simulink model "VectorControl002"  (R2018a)
settings: Solver=ode15s  StartTime=0  StopTime=1  FixedStep=0.001  MaxStep=1e-4  RelTol=1e-6  AbsTol=1e-6  EnableMultiTasking=on
PreLoadFcn:
  | Param000
StopFcn:
  | % TNAnalyzexxxPlot
values from neighbouring files (symbols this model uses):
  DCVoltage = 100    [Param000.m]    (also in StartSim.m; StartSim_NoNoise.m)
  MotInertia = 10*rand()*1e-3    [Param000.m]    (also in StartSim.m = 0.1*rand()*1e-3; StartSim_NoNoise.m = 0.1*rand()*1e-3)
  MotPhaseL = 0.01 + 100 * rand()    [Param000.m]    (also in StartSim.m = (0.001 + 10 * rand())*1e-3; StartSim_NoNoise.m = (0.001 + 10 * rand())*1e-3)
  MotPhaseR = 0.01 + 100 * rand()    [Param000.m]    (also in StartSim.m = 0.001 + 10 * rand(); StartSim_NoNoise.m = 0.001 + 10 * rand())
  MotPole = 20    [Param000.m]    (also in StartSim.m = 1; StartSim_NoNoise.m = 1)
  MotVisco = rand()*1e-6    [Param000.m]    (also in StartSim.m = 0.01*rand()*1e-6; StartSim_NoNoise.m = 0.01*rand()*1e-6)
  Ts = 1e-6    (= 1e-06)    [StartSim.m]    (also in StartSim_NoNoise.m)
undefined symbols (not defined in the file or in its folder): AmpCap, AmpCapR, MotLineR, PowerLineR
libraries: powerlib x43, simulink x2, powerlib_meascontrol x2, pePwmGeneratorTwoLevel x1
Description:
  | This example illustrates use of the BLDC in a closed-loop
  | speed and voltage control on a 1 kW, 3000 rpm industrial motor
  | 
  | 
  | Copyright 2008-2017 The MathWorks, Inc.
settings Model: ExtModeAutoUpdateStatusClock=off  Creator=MathWorks  LastModifiedBy=1468993
settings SolverCC: AutoScaleAbsTol=off  MaxConsecutiveZCs=10000  ZeroCrossAlgorithm=Adaptive  DecoupledContinuousIntegration=on
settings DataIOCC: Decimation=100  SaveFormat=Array  ReturnWorkspaceOutputs=on  SignalLoggingName=sigsOut
settings OptimizationCC: DefaultParameterBehavior=Inlined  UseDivisionForNetSlopeComputation=on  UseFloatMulNetSlope=on  InlineInvariantSignals=on  PassReuseOutputArgsAs=Individual arguments  ExpressionDepthLimit=2147483647  ZeroExternalMemoryAtStartup=off  ZeroInternalMemoryAtStartup=off  NoFixptDivByZeroProtection=on  EfficientFloat2IntCast=on  LifeSpan=1  OptimizeDataStoreBuffers=off  BusAssignmentInplaceUpdate=off  OptimizationLevel=level0
settings DebuggingCC: AlgebraicLoopMsg=none  UnderspecifiedInitializationDetection=Classic  MergeDetectMultiDrivingBlocksExec=none  SignalResolutionControl=TryResolveAllWithWarning  MultiTaskDSMMsg=warning  MultiTaskCondExecSysMsg=none  ParameterTunabilityLossMsg=error  FcnCallInpInsideContextMsg=warning  StateNameClashWarn=warning  SFUnexpectedBacktrackingDiag=warning  SFNoUnconditionalDefaultTransitionDiag=warning  SFExecutionAtInitializationDiag=none
settings HardwareCC: ProdBitPerPointer=32  ProdBitPerSizeT=32  ProdBitPerPtrDiffT=32  ProdLargestAtomicInteger=Long  ProdWordSize=32  ProdLongLongMode=on  ProdHWDeviceType=ARM Compatible->ARM 10  TargetUnknown=on
settings ModelReferenceCC: PropagateSignalLabelsOutOfModel=off
settings SFSimCC: MATLABDynamicMemAlloc=off
settings RTWCC: SystemTargetFile=ert.tlc  TemplateMakefile=ert_default_tmf  GenerateReport=on  IncludeHyperlinkInReport=on  LaunchReport=on  GenerateTraceInfo=on  GenerateTraceReport=on  GenerateTraceReportSl=on  GenerateTraceReportSf=on  GenerateTraceReportEml=on  GenerateCodeMetricsReport=on
settings CodeAppCC: ForceParamTrailComments=on  IgnoreCustomStorageClasses=off  OperatorAnnotations=on  SimulinkDataObjDesc=on  SFDataObjDesc=on  CustomSymbolStrGlobalVar=rt$N$M  CustomSymbolStrType=$N$M  CustomSymbolStrFcn=$N$M$F  CustomSymbolStrMacro=$N$M  InsertBlockDesc=on
settings ERTTargetCC: GenerateSampleERTMain=on  IncludeMdlTerminateFcn=off  CombineSignalStateStructs=on  SupportComplex=off  SupportContinuousTime=on  SupportNonInlinedSFcns=on  InlinedParameterPlacement=NonHierarchical  ERTCustomFileTemplate=example_file_process.tlc  ERTFilePackagingFormat=CompactWithDataFile
settings ConfigComp: CovMetricSettings=dw  CovHtmlReporting=on  CovSaveCumulativeToWorkspaceVar=on  CovSaveSingleToWorkspaceVar=on  CovExternalEMLEnable=off  CovSFcnEnable=off
settings SimscapeCC: SimscapeNormalizeSystem=off

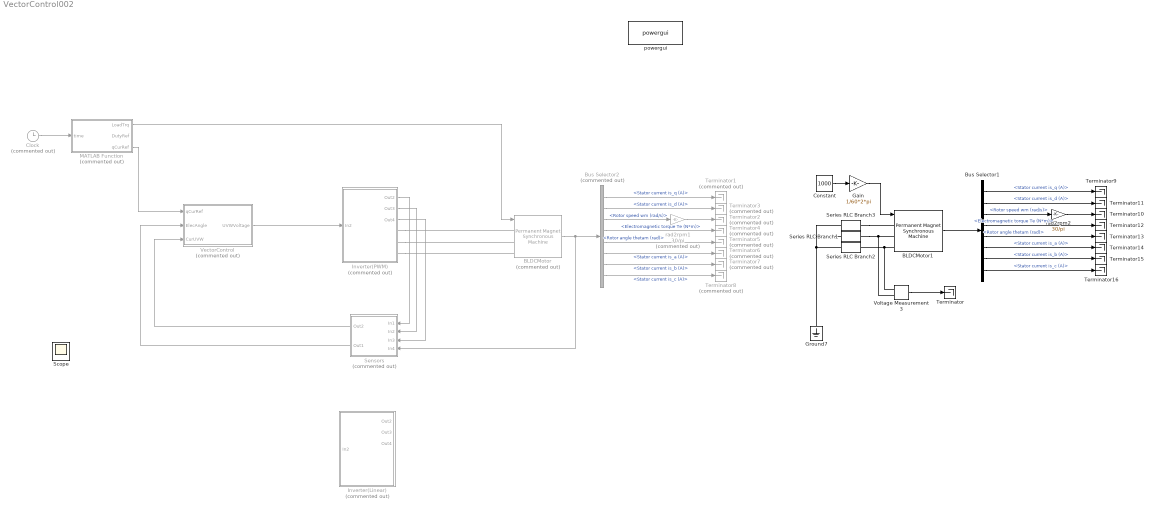
== system VectorControl002 ==
  BLDCMotor : powerlib/Machines/Permanent Magnet Synchronous Machine  Commented=on  NbPhases=3  FluxDistribution=Sinusoidal  RotorType=Round  MechanicalLoad=Torque Tm  PresetModel=No  ShowDetailedParameters=on  MeasurementBus=off  Resistance=MotPhaseR  Inductance=MotPhaseL  dqInductances=[8.5e-3, 8.5e-3]  La=MotPhaseL  MachineConstant=Voltage Constant (V_peak L-L / krpm)  Flux=0.01021  VoltageCst=MotVoltageConst  TorqueCst=0.30629  Flat=120  Mechanical=[MotInertia MotVisco MotPole 0]  PolePairs=20  InitialConditions=[0,0, 0,0]  InitialConditions5ph=[0 0 0 0 0 0]  TsPowergui=0  TsBlock=-1  RefAngle=90 degrees behind phase A axis (modified Park)
      settings: SourceProductName=Simscape Power Systems
  BLDCMotor1 : powerlib/Machines/Permanent Magnet Synchronous Machine  NbPhases=3  FluxDistribution=Sinusoidal  RotorType=Round  MechanicalLoad=Speed w  PresetModel=No  ShowDetailedParameters=on  MeasurementBus=off  Resistance=MotPhaseR  Inductance=MotPhaseL  dqInductances=[8.5e-3, 8.5e-3]  La=MotPhaseL  MachineConstant=Voltage Constant (V_peak L-L / krpm)  Flux=0.01021  VoltageCst=MotVoltageConst  TorqueCst=0.30629  Flat=120  Mechanical=[MotInertia MotVisco MotPole 0]  PolePairs=20  InitialConditions=[0,0, 0,0]  InitialConditions5ph=[0 0 0 0 0 0]  TsPowergui=0  TsBlock=-1  RefAngle=90 degrees behind phase A axis (modified Park)
      settings: SourceProductName=Simscape Power Systems
  Bus Selector1 : BusSelector  OutputSignals=Stator current is_q (A),Stator current is_d (A),Rotor speed wm (rad/s),Electromagnetic torque Te (N*m),Rotor angle thetam (rad),Stator current is_a (A),Stator current is_b (A),Stator current is_c (A)
  Bus Selector2 : BusSelector  Commented=on  OutputSignals=Stator current is_q (A),Stator current is_d (A),Rotor speed wm (rad/s),Electromagnetic torque Te (N*m),Rotor angle thetam (rad),Stator current is_a (A),Stator current is_b (A),Stator current is_c (A)
  Clock : Clock  Commented=on
  Constant : Constant  Value=1000
  Gain : Gain  Gain=1/60*2*pi
  Ground7 : powerlib/Elements/Ground  LConnTagsString=a
  Inverter(Linear) : Subsystem  Commented=on
  Inverter(PWM) : Subsystem  Commented=on
  MATLAB Function : MATLAB Function  Commented=on  TreatAsAtomicUnit=on
  Sensors : Subsystem  Commented=on
  Series RLC Branch1 : powerlib/Elements/Series RLC Branch  LConnTagsString=__new0  RConnTagsString=__new0  BranchType=R  Resistance=1e6  Inductance=1e-3  SetiL0=off  InitialCurrent=0  Capacitance=100e-6  Setx0=on  InitialVoltage=3.7*7*3  Measurements=None
  Series RLC Branch2 : powerlib/Elements/Series RLC Branch  LConnTagsString=__new0  RConnTagsString=__new0  BranchType=R  Resistance=1e6  Inductance=1e-3  SetiL0=off  InitialCurrent=0  Capacitance=100e-6  Setx0=on  InitialVoltage=3.7*7*3  Measurements=None
  Series RLC Branch3 : powerlib/Elements/Series RLC Branch  LConnTagsString=__new0  RConnTagsString=__new0  BranchType=R  Resistance=1e6  Inductance=1e-3  SetiL0=off  InitialCurrent=0  Capacitance=100e-6  Setx0=on  InitialVoltage=3.7*7*3  Measurements=None
  Terminator{,9..16} (9 alike) : Terminator
  Terminator{1..8} (8 alike) : Terminator  Commented=on
  VectorControl : Subsystem  Commented=on
  Voltage Measurement3 : powerlib/Measurements/Voltage Measurement  PhasorSimulation=off  OutputType=Complex  PSBequivalent=0
  powergui : powerlib/powergui  Priority=2  SimulationMode=Continuous  SampleTime=Ts  frequency=60  Iterations=50  frequencyindice=0  Pbase=100e6  ErrMax=1e-4  UnitsV=kV  UnitsW=MW  buscounter=0  FunctionMessages=off  echomessages=off  EnableUseOfTLC=off  CurrentSourceSwitches=off  DisableSnubberDevices=off  DisableRonSwitches=off  DisableVfSwitches=off  DisplayEquations=off  SolverType=Tustin/Backward Euler (TBE)  Interpol=off  ExternalGateDelay=off  methode=off  Ts=100  x0status=blocks  SPID=off  SwTol=0  HookPort=off  RestoreLinks=warning  ResistiveCurrentMeasurement=off  Frange=[0:2:500]  Ylog=off  Xlog=on  ShowGrid=off  save=off  variable=ZData  structure=0  ZoomFFT=on  StartTime=0.0  cycles=1  DisplayStyle=1  fundamental=60  FreqAxis=off  MaxFrequency=1000  frequencyindicesteady=1  RmsSteady=1  display=off
  rad2rpm1 : Gain  Commented=on  Gain=30/pi
  rad2rpm2 : Gain  Gain=30/pi
  Scope : Scope
  wires:
  Clock/1 -> MATLAB Function/1(time)
  Bus Selector2/3 -> rad2rpm1/1  "<Rotor speed wm (rad/s)>"
  MATLAB Function/1(LoadTrq) -> BLDCMotor/1
  BLDCMotor/1 -> Sensors/4(In4), Bus Selector2/1
  MATLAB Function/3(qCurRef) -> VectorControl/1(qCurRef)
  rad2rpm1/1 -> Terminator2/1
  Bus Selector2/1 -> Terminator1/1  "<Stator current is_q (A)>"
  Bus Selector2/2 -> Terminator3/1  "<Stator current is_d (A)>"
  Bus Selector2/4 -> Terminator4/1  "<Electromagnetic torque Te (N*m)>"
  Bus Selector2/5 -> Terminator5/1  "<Rotor angle thetam (rad)>"
  Bus Selector2/6 -> Terminator6/1  "<Stator current is_a (A)>"
  Bus Selector2/7 -> Terminator7/1  "<Stator current is_b (A)>"
  Bus Selector2/8 -> Terminator8/1  "<Stator current is_c (A)>"
  Inverter(PWM)/1(Out2) -> Sensors/1(In1)
  Inverter(PWM)/2(Out3) -> Sensors/2(In2)
  Inverter(PWM)/3(Out4) -> Sensors/3(In3)
  VectorControl/1(UVWVoltage) -> Inverter(PWM)/1(In2)
  Sensors/1(Out2) -> VectorControl/3(CurUVW)
  Sensors/2(Out1) -> VectorControl/2(ElecAngle)
  Bus Selector1/8 -> Terminator16/1  "<Stator current is_c (A)>"
  Bus Selector1/7 -> Terminator15/1  "<Stator current is_b (A)>"
  Bus Selector1/6 -> Terminator14/1  "<Stator current is_a (A)>"
  Bus Selector1/5 -> Terminator13/1  "<Rotor angle thetam (rad)>"
  Bus Selector1/4 -> Terminator12/1  "<Electromagnetic torque Te (N*m)>"
  Bus Selector1/2 -> Terminator11/1  "<Stator current is_d (A)>"
  Bus Selector1/1 -> Terminator9/1  "<Stator current is_q (A)>"
  rad2rpm2/1 -> Terminator10/1
  BLDCMotor1/1 -> Bus Selector1/1
  Bus Selector1/3 -> rad2rpm2/1  "<Rotor speed wm (rad/s)>"
  Constant/1 -> Gain/1
  Gain/1 -> BLDCMotor1/1
  Voltage Measurement3/1 -> Terminator/1
  connections:
  Inverter(PWM)/RConn2 -- BLDCMotor/LConn2
  Inverter(PWM)/RConn3 -- BLDCMotor/LConn3
  Inverter(PWM)/RConn1 -- BLDCMotor/LConn1
  Series RLC Branch3/LConn1 -- BLDCMotor1/LConn1
  Series RLC Branch1/LConn1 -- Voltage Measurement3/LConn2 -- BLDCMotor1/LConn2
  BLDCMotor1/LConn3 -- Series RLC Branch2/LConn1 -- Voltage Measurement3/LConn1
  Ground7/LConn1 -- Series RLC Branch1/RConn1 -- Series RLC Branch3/RConn1 -- Series RLC Branch2/RConn1

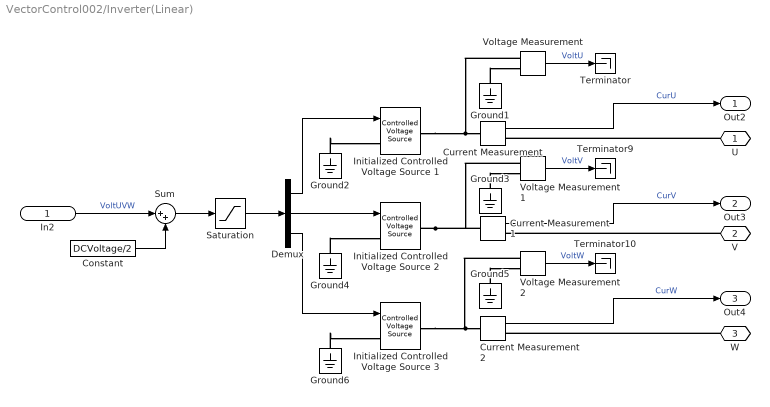
== system VectorControl002/Inverter(Linear) ==
  In2 : Inport
  Constant : Constant  Value=DCVoltage/2
  Current Measurement : powerlib/Measurements/Current Measurement  PhasorSimulation=off  OutputType=Complex  PSBequivalent=0
  Current Measurement1 : powerlib/Measurements/Current Measurement  PhasorSimulation=off  OutputType=Complex  PSBequivalent=0
  Current Measurement2 : powerlib/Measurements/Current Measurement  PhasorSimulation=off  OutputType=Complex  PSBequivalent=0
  Demux : Demux  Outputs=3
  Ground{1..6} (6 alike) : powerlib/Elements/Ground  LConnTagsString=a
  Initialized Controlled Voltage Source 1 : powerlib/Electrical Sources/Controlled Voltage Source  Description=source block  Initialize=off  Source_Type=DC  Amplitude=120  Phase=0  Frequency=60  Measurements=None
      settings: AttributesFormatString=\n
  Initialized Controlled Voltage Source 2 : powerlib/Electrical Sources/Controlled Voltage Source  Description=source block  Initialize=off  Source_Type=DC  Amplitude=120  Phase=0  Frequency=60  Measurements=None
      settings: AttributesFormatString=\n
  Initialized Controlled Voltage Source 3 : powerlib/Electrical Sources/Controlled Voltage Source  Description=source block  Initialize=off  Source_Type=DC  Amplitude=120  Phase=0  Frequency=60  Measurements=None
      settings: AttributesFormatString=\n
  Saturation : Saturate  UpperLimit=DCVoltage  LowerLimit=0
  Sum : Sum  Inputs=|++
  Terminator : Terminator
  Terminator10 : Terminator
  Terminator9 : Terminator
  Voltage Measurement : powerlib/Measurements/Voltage Measurement  PhasorSimulation=off  OutputType=Complex  PSBequivalent=0
  Voltage Measurement1 : powerlib/Measurements/Voltage Measurement  PhasorSimulation=off  OutputType=Complex  PSBequivalent=0
  Voltage Measurement2 : powerlib/Measurements/Voltage Measurement  PhasorSimulation=off  OutputType=Complex  PSBequivalent=0
  U : PMIOPort  Side=Right
  V : PMIOPort  Port=2  Side=Right
  W : PMIOPort  Port=3  Side=Right
  Out2 : Outport
  Out3 : Outport  Port=2
  Out4 : Outport  Port=3
  wires:
  Voltage Measurement1/1 -> Terminator9/1  "VoltV"
  Voltage Measurement2/1 -> Terminator10/1  "VoltW"
  Demux/3 -> Initialized Controlled Voltage Source 3/1
  Voltage Measurement/1 -> Terminator/1  "VoltU"
  Demux/2 -> Initialized Controlled Voltage Source 2/1
  Demux/1 -> Initialized Controlled Voltage Source 1/1
  Current Measurement1/1 -> Out3/1  "CurV"
  Current Measurement2/1 -> Out4/1  "CurW"
  Current Measurement/1 -> Out2/1  "CurU"
  In2/1 -> Sum/1  "VoltUVW"
  Constant/1 -> Sum/2
  Sum/1 -> Saturation/1
  Saturation/1 -> Demux/1
  connections:
  Initialized Controlled Voltage Source 1/RConn1 -- Current Measurement/LConn1 -- Voltage Measurement/LConn1
  Current Measurement2/LConn1 -- Initialized Controlled Voltage Source 3/RConn1 -- Voltage Measurement2/LConn1
  Initialized Controlled Voltage Source 2/RConn1 -- Current Measurement1/LConn1 -- Voltage Measurement1/LConn1
  Ground1/LConn1 -- Voltage Measurement/LConn2
  Ground3/LConn1 -- Voltage Measurement1/LConn2
  Ground6/LConn1 -- Initialized Controlled Voltage Source 3/LConn1
  Ground2/LConn1 -- Initialized Controlled Voltage Source 1/LConn1
  U/RConn1 -- Current Measurement/RConn1
  Ground5/LConn1 -- Voltage Measurement2/LConn2
  Ground4/LConn1 -- Initialized Controlled Voltage Source 2/LConn1
  W/RConn1 -- Current Measurement2/RConn1
  V/RConn1 -- Current Measurement1/RConn1

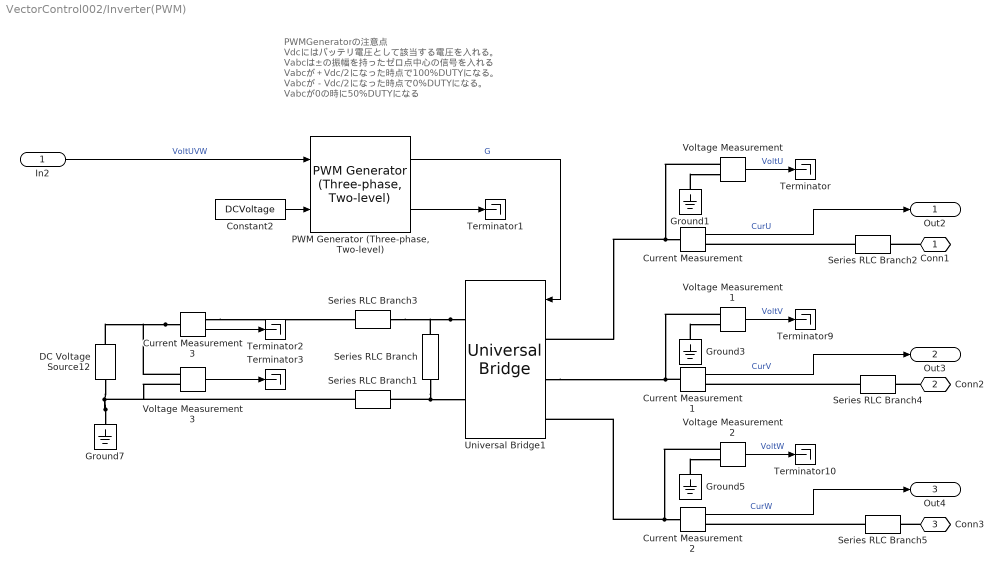
== system VectorControl002/Inverter(PWM) ==
  note: PWMGeneratorの注意点
      | Vdcにはバッテリ電圧として該当する電圧を入れる。
      | Vabcは±の振幅を持ったゼロ点中心の信号を入れる
      | Vabcが＋Vdc/2になった時点で100%DUTYになる。
      | Vabcが－Vdc/2になった時点で0%DUTYになる。
      | Vabcが0の時に50%DUTYになる
  In2 : Inport
  Constant2 : Constant  Value=DCVoltage
  Current Measurement{,1..3} (4 alike) : powerlib/Measurements/Current Measurement  PhasorSimulation=off  OutputType=Complex  PSBequivalent=0
  DC Voltage Source12 : powerlib/Electrical Sources/DC Voltage Source  Amplitude=DCVoltage  Measurements=None
  Ground{1,3,5,7} (4 alike) : powerlib/Elements/Ground  LConnTagsString=a
  "PWM Generator (Three-phase, Two-level)" : pePwmGeneratorTwoLevel/PWM Generator (Three-phase, Two-level)  OverrideUsingVariant=NaturalMode  PWMMode=Continuous PWM (CPWM)  CPWMMode=SPWM: sinusoidal PWM  DPWMMode=60 DPWM: 60 degree discontinuous PWM  fsw=AmpCarryFreq  Ts=1e-6
      settings: SamplingMode=Natural
  Series RLC Branch : powerlib/Elements/Series RLC Branch  LConnTagsString=__new0  RConnTagsString=__new0  BranchType=RC  Resistance=AmpCapR/10  Inductance=1e-3  SetiL0=off  InitialCurrent=0  Capacitance=AmpCap  Setx0=on  InitialVoltage=AmpCapV  Measurements=None
  Series RLC Branch1 : powerlib/Elements/Series RLC Branch  LConnTagsString=__new0  RConnTagsString=__new0  BranchType=R  Resistance=PowerLineR  Inductance=1e-3  SetiL0=off  InitialCurrent=0  Capacitance=100e-6  Setx0=on  InitialVoltage=3.7*7*3  Measurements=None
  Series RLC Branch2 : powerlib/Elements/Series RLC Branch  LConnTagsString=__new0  RConnTagsString=__new0  BranchType=R  Resistance=MotLineR  Inductance=1e-3  SetiL0=off  InitialCurrent=0  Capacitance=1e-6  Setx0=off  InitialVoltage=0  Measurements=None
  Series RLC Branch3 : powerlib/Elements/Series RLC Branch  LConnTagsString=__new0  RConnTagsString=__new0  BranchType=R  Resistance=PowerLineR  Inductance=1e-3  SetiL0=off  InitialCurrent=0  Capacitance=100e-6  Setx0=on  InitialVoltage=3.7*7*3  Measurements=None
  Series RLC Branch4 : powerlib/Elements/Series RLC Branch  LConnTagsString=__new0  RConnTagsString=__new0  BranchType=R  Resistance=MotLineR  Inductance=1e-3  SetiL0=off  InitialCurrent=0  Capacitance=1e-6  Setx0=off  InitialVoltage=0  Measurements=None
  Series RLC Branch5 : powerlib/Elements/Series RLC Branch  LConnTagsString=__new0  RConnTagsString=__new0  BranchType=R  Resistance=MotLineR  Inductance=1e-3  SetiL0=off  InitialCurrent=0  Capacitance=1e-6  Setx0=off  InitialVoltage=0  Measurements=None
  Terminator{,1..3,9..10} (6 alike) : Terminator
  Universal Bridge1 : powerlib/Power Electronics/Universal Bridge  Arms=3  SnubberResistance=1e5  SnubberCapacitance=inf  Device=MOSFET / Diodes  Ron=1e-6  Lon=0  ForwardVoltages="[  0  0  ]"  ForwardVoltage=0  GTOparameters=[ 10e-6 , 20e-6 ]  IGBTparameters=[ 1e-6 , 2e-6 ]  Measurements=None  Measurements_2=None  converterType=Rectifier
  Voltage Measurement{,1..3} (4 alike) : powerlib/Measurements/Voltage Measurement  PhasorSimulation=off  OutputType=Complex  PSBequivalent=0
  Conn1 : PMIOPort  Side=Right
  Conn2 : PMIOPort  Port=2  Side=Right
  Conn3 : PMIOPort  Port=3  Side=Right
  Out2 : Outport
  Out3 : Outport  Port=2
  Out4 : Outport  Port=3
  wires:
  Voltage Measurement1/1 -> Terminator9/1  "VoltV"
  Voltage Measurement2/1 -> Terminator10/1  "VoltW"
  Voltage Measurement/1 -> Terminator/1  "VoltU"
  Current Measurement1/1 -> Out3/1  "CurV"
  Current Measurement2/1 -> Out4/1  "CurW"
  Current Measurement/1 -> Out2/1  "CurU"
  Current Measurement3/1 -> Terminator2/1
  Voltage Measurement3/1 -> Terminator3/1
  Constant2/1 -> "PWM Generator (Three-phase, Two-level)"/2
  "PWM Generator (Three-phase, Two-level)"/1 -> Universal Bridge1/1  "G"
  "PWM Generator (Three-phase, Two-level)"/2 -> Terminator1/1
  In2/1 -> "PWM Generator (Three-phase, Two-level)"/1  "VoltUVW"
  connections:
  Voltage Measurement/LConn1 -- Current Measurement/LConn1 -- Universal Bridge1/LConn1
  Voltage Measurement2/LConn1 -- Current Measurement2/LConn1 -- Universal Bridge1/LConn3
  Current Measurement1/LConn1 -- Voltage Measurement1/LConn1 -- Universal Bridge1/LConn2
  Ground1/LConn1 -- Voltage Measurement/LConn2
  Ground3/LConn1 -- Voltage Measurement1/LConn2
  Series RLC Branch2/LConn1 -- Current Measurement/RConn1
  Ground5/LConn1 -- Voltage Measurement2/LConn2
  Series RLC Branch5/LConn1 -- Current Measurement2/RConn1
  Series RLC Branch4/LConn1 -- Current Measurement1/RConn1
  Current Measurement3/LConn1 -- Voltage Measurement3/LConn1 -- DC Voltage Source12/RConn1
  Ground7/LConn1 -- Voltage Measurement3/LConn2 -- Series RLC Branch1/RConn1 -- DC Voltage Source12/LConn1
  Universal Bridge1/RConn1 -- Series RLC Branch/LConn1 -- Series RLC Branch3/LConn1
  Series RLC Branch/RConn1 -- Universal Bridge1/RConn2 -- Series RLC Branch1/LConn1
  Current Measurement3/RConn1 -- Series RLC Branch3/RConn1
  Conn1/RConn1 -- Series RLC Branch2/RConn1
  Conn2/RConn1 -- Series RLC Branch4/RConn1
  Conn3/RConn1 -- Series RLC Branch5/RConn1

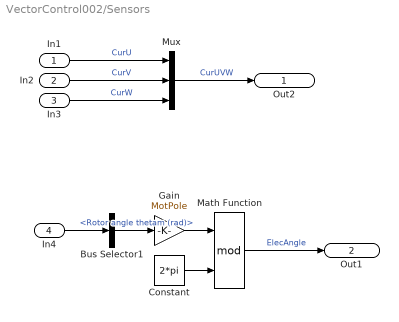
== system VectorControl002/Sensors ==
  In1 : Inport
  In2 : Inport  Port=2
  In3 : Inport  Port=3
  In4 : Inport  Port=4
  Bus Selector1 : BusSelector  OutputSignals=Rotor angle thetam (rad)
  Constant : Constant  Value=2*pi
  Gain : Gain  Gain=MotPole
  Math Function : Math  Operator=mod  SaturateOnIntegerOverflow=on
  Mux : Mux  Inputs=3
  Out2 : Outport
  Out1 : Outport  Port=2
  wires:
  Gain/1 -> Math Function/1
  Bus Selector1/1 -> Gain/1  "<Rotor angle thetam (rad)>"
  In3/1 -> Mux/3  "CurW"
  In1/1 -> Mux/1  "CurU"
  In4/1 -> Bus Selector1/1
  Constant/1 -> Math Function/2
  In2/1 -> Mux/2  "CurV"
  Math Function/1 -> Out1/1  "ElecAngle"
  Mux/1 -> Out2/1  "CurUVW"

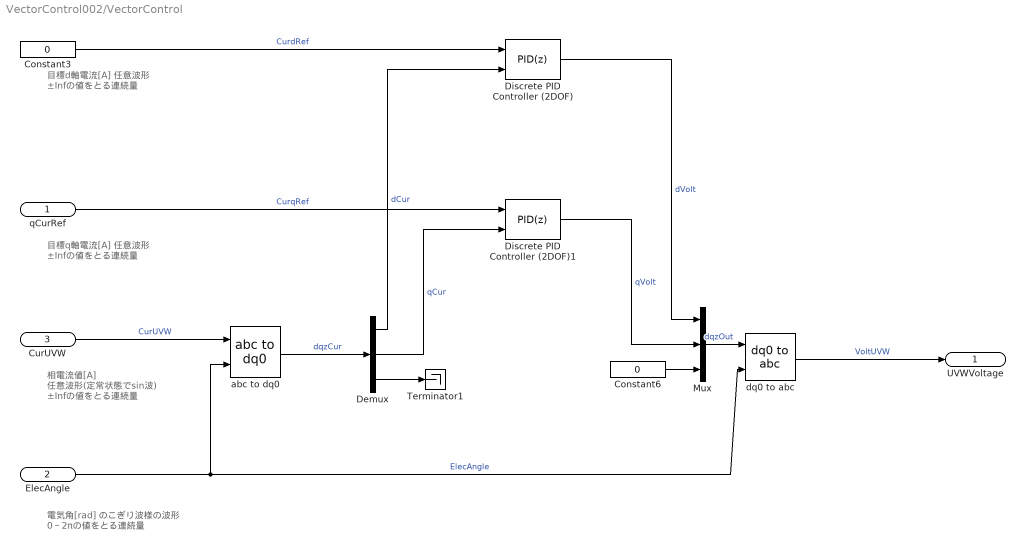
== system VectorControl002/VectorControl ==
  note: 電気角[rad]
      | のこぎり波様の波形
      | 0～2πの値をとる連続量
  note: 相電流値[A]
      | 任意波形(定常状態でsin波)
      | ±Infの値をとる連続量
  note: 目標q軸電流[A]
      | 任意波形
      | ±Infの値をとる連続量
  note: 目標d軸電流[A]
      | 任意波形
      | ±Infの値をとる連続量
  qCurRef : Inport
  ElecAngle : Inport  Port=2
  CurUVW : Inport  Port=3
  Constant3 : Constant  Value=0
  Constant6 : Constant  Value=0
  Demux : Demux  Outputs=3
  Discrete PID Controller (2DOF) : simulink/Continuous/PID Controller (2DOF)  Controller=PID  TimeDomain=Discrete-time  SampleTime=50e-6  IntegratorMethod=Forward Euler  FilterMethod=Forward Euler  Form=Parallel  UseFilter=on  ControllerParametersSource=internal  P=0.0463529010923698  I=32.9269944116698  D=4.2169419182621e-06  N=1663.51306055894  b=1  c=1  InitialConditionSource=internal  InitialConditionForIntegrator=0  InitialConditionForFilter=0  ExternalReset=none  LimitOutput=on  UpperSaturationLimit=DCVoltage  LowerSaturationLimit=-DCVoltage  LinearizeAsGain=off  AntiWindupMode=clamping  Kb=1  TrackingMode=off  Kt=1  PParamMin=[]  PParamMax=[]  IParamMin=[]  IParamMax=[]  DParamMin=[]  DParamMax=[]  NParamMin=[]  NParamMax=[]  bParamMin=[]  bParamMax=[]  cParamMin=[]  cParamMax=[]  KbParamMin=[]  KbParamMax=[]  KtParamMin=[]  KtParamMax=[]  POutMin=[]  POutMax=[]  IOutMin=[]  IOutMax=[]  DOutMin=[]  DOutMax=[]  NOutMin=[]  NOutMax=[]  bOutMin=[]  bOutMax=[]  cOutMin=[]  cOutMax=[]  KbOutMin=[]  KbOutMax=[]  KtOutMin=[]  KtOutMax=[]  IntegratorOutMin=[]  IntegratorOutMax=[]  FilterOutMin=[]  FilterOutMax=[]  SumOutMin=[]  SumOutMax=[]  Sum1OutMin=[]  Sum1OutMax=[]  Sum2OutMin=[]  Sum2OutMax=[]  Sum3OutMin=[]  Sum3OutMax=[]  SumI1OutMin=[]  SumI1OutMax=[]  SumI2OutMin=[]  SumI2OutMax=[]  SumI3OutMin=[]  SumI3OutMax=[]  SumDOutMin=[]  SumDOutMax=[]  SaturationOutMin=[]  SaturationOutMax=[]  IntegratorContinuousStateAttributes=''  IntegratorStateMustResolveToSignalObject=off  IntegratorRTWStateStorageClass=Auto  FilterContinuousStateAttributes=''  FilterStateMustResolveToSignalObject=off  FilterRTWStateStorageClass=Auto  DifferentiatorICPrevScaledInput=0  DifferentiatorOutMin=[]  DifferentiatorOutMax=[]  FilterDiffOutCoefMin=[]  FilterDiffOutCoefMax=[]  SumDenOutMin=[]  SumDenOutMax=[]  SumNumOutMin=[]  SumNumOutMax=[]  ReciprocalOutMin=[]  ReciprocalOutMax=[]  DivideOutMin=[]  DivideOutMax=[]  TunerSelectOption=Transfer Function Based (PID Tuner App)
  Discrete PID Controller (2DOF)1 : simulink/Continuous/PID Controller (2DOF)  Controller=PID  TimeDomain=Discrete-time  SampleTime=50e-6  IntegratorMethod=Forward Euler  FilterMethod=Forward Euler  Form=Parallel  UseFilter=on  ControllerParametersSource=internal  P=0.0463529010923698  I=32.9269944116698  D=4.2169419182621e-06  N=1663.51306055894  b=1  c=1  InitialConditionSource=internal  InitialConditionForIntegrator=0  InitialConditionForFilter=0  ExternalReset=none  ZeroCross=off  LimitOutput=on  UpperSaturationLimit=DCVoltage  LowerSaturationLimit=-DCVoltage  LinearizeAsGain=off  AntiWindupMode=clamping  Kb=1  TrackingMode=off  Kt=1  PParamMin=[]  PParamMax=[]  IParamMin=[]  IParamMax=[]  DParamMin=[]  DParamMax=[]  NParamMin=[]  NParamMax=[]  bParamMin=[]  bParamMax=[]  cParamMin=[]  cParamMax=[]  KbParamMin=[]  KbParamMax=[]  KtParamMin=[]  KtParamMax=[]  POutMin=[]  POutMax=[]  IOutMin=[]  IOutMax=[]  DOutMin=[]  DOutMax=[]  NOutMin=[]  NOutMax=[]  bOutMin=[]  bOutMax=[]  cOutMin=[]  cOutMax=[]  KbOutMin=[]  KbOutMax=[]  KtOutMin=[]  KtOutMax=[]  IntegratorOutMin=[]  IntegratorOutMax=[]  FilterOutMin=[]  FilterOutMax=[]  SumOutMin=[]  SumOutMax=[]  Sum1OutMin=[]  Sum1OutMax=[]  Sum2OutMin=[]  Sum2OutMax=[]  Sum3OutMin=[]  Sum3OutMax=[]  SumI1OutMin=[]  SumI1OutMax=[]  SumI2OutMin=[]  SumI2OutMax=[]  SumI3OutMin=[]  SumI3OutMax=[]  SumDOutMin=[]  SumDOutMax=[]  SaturationOutMin=[]  SaturationOutMax=[]  IntegratorContinuousStateAttributes=''  IntegratorStateMustResolveToSignalObject=off  IntegratorRTWStateStorageClass=Auto  FilterContinuousStateAttributes=''  FilterStateMustResolveToSignalObject=off  FilterRTWStateStorageClass=Auto  DifferentiatorICPrevScaledInput=0  DifferentiatorOutMin=[]  DifferentiatorOutMax=[]  FilterDiffOutCoefMin=[]  FilterDiffOutCoefMax=[]  SumDenOutMin=[]  SumDenOutMax=[]  SumNumOutMin=[]  SumNumOutMax=[]  ReciprocalOutMin=[]  ReciprocalOutMax=[]  DivideOutMin=[]  DivideOutMax=[]  TunerSelectOption=Transfer Function Based (PID Tuner App)
  Mux : Mux  Inputs=3
  Terminator1 : Terminator
  abc to dq0 : powerlib_meascontrol/Transformations/abc to dq0  Alignment=90 degrees behind phase A axis
  dq0 to abc : powerlib_meascontrol/Transformations/dq0 to abc  Alignment=90 degrees behind phase A axis
  UVWVoltage : Outport
  wires:
  ElecAngle/1 -> dq0 to abc/2, abc to dq0/2  "ElecAngle"
  dq0 to abc/1 -> UVWVoltage/1  "VoltUVW"
  abc to dq0/1 -> Demux/1  "dqzCur"
  Mux/1 -> dq0 to abc/1  "dqzOut"
  Constant6/1 -> Mux/3
  Demux/3 -> Terminator1/1
  CurUVW/1 -> abc to dq0/1  "CurUVW"
  Demux/1 -> Discrete PID Controller (2DOF)/2  "dCur"
  Discrete PID Controller (2DOF)/1 -> Mux/1  "dVolt"
  Constant3/1 -> Discrete PID Controller (2DOF)/1  "CurdRef"
  qCurRef/1 -> Discrete PID Controller (2DOF)1/1  "CurqRef"
  Discrete PID Controller (2DOF)1/1 -> Mux/2  "qVolt"
  Demux/2 -> Discrete PID Controller (2DOF)1/2  "qCur"

== matlab function VectorControl002/MATLAB Function ==
  data: LoadTrq output; time input; DutyRef output; qCurRef output
function [LoadTrq,DutyRef,qCurRef] = fcn(time)

%初期化していない変数の参照を避けるため出力変数には必ず1回は値を代入する
DutyRef = 0;
qCurRef = 0;
LoadTrq = 0;

%最終到達DUTY
DutyGoal = 1;
%到達時刻
DutyGoalTime = 0.1;
%DUTYの上昇率
DutyRate = DutyGoal / DutyGoalTime;

%加速中であればStableGoalTimeの時間を後ろにずらす(加算値を増やす)
StableGoalTime = DutyGoalTime + 0.1;

%最終到達負荷トルク
TrqGoal = 50;
%シミュレーションが1秒で終わる前提で、0.95秒で80Nmに達するようにする
TrqGoalTime = 0.95;
%負荷トルクの上昇率
TrqRate = TrqGoal / (TrqGoalTime - StableGoalTime);

%ランプ状にDUTYを上げていく区間
if (0 < time) && (time <= DutyGoalTime)
    DutyRef = DutyRate * time; %時間経過に伴ってDUTYを増やす
    qCurRef = 1;
    LoadTrq = 0;
else
    %最終DUTYに到達して安定している区間
    if (DutyGoalTime < time) && (time <= StableGoalTime)
        DutyRef = DutyGoal;
        qCurRef = 0;
        LoadTrq = 0;
    else
        %負荷トルクをかける区間
        if (StableGoalTime < time) && (time <= TrqGoalTime)
            DutyRef = DutyGoal;
            LoadTrq = TrqRate * (time - StableGoalTime);
            qCurRef = 15*LoadTrq;
        else
            if (TrqGoalTime < time)
                DutyRef = DutyGoal;
                LoadTrq = TrqGoal;                
                qCurRef = 15*LoadTrq;
            end
        end
    end    
end
